simulink model "AlphaIntegrator"  (Simulink 6.6)
settings: Solver=ode45  StartTime=0.0  StopTime=10.0  RelTol=1e-3
values from neighbouring files (symbols this model uses):
  steps = length(canoga_deltaT10)    [CR_init_setup.m]
undefined symbols (not defined in the file or in its folder): alpha, beta, deltat, gamma, iterations
settings Model: Creator=Tommy  LastModifiedBy=Tommy

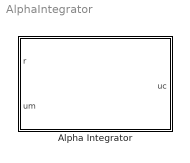
== system AlphaIntegrator ==
  Alpha Integrator : Subsystem
      mask Type: Apha Method with Fixed Number of Iterations
      mask Description: Apha Method with Fixed Number of Iterations

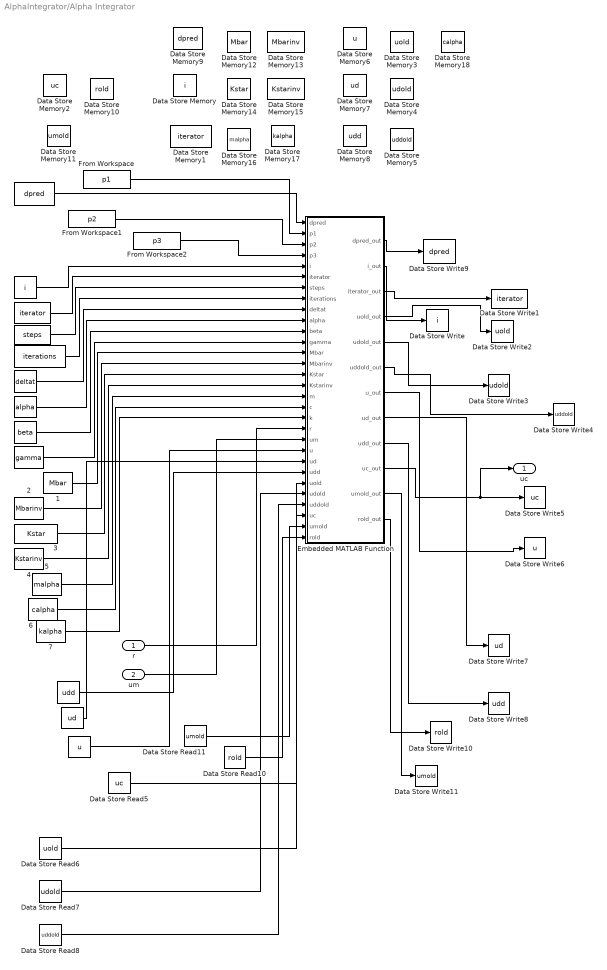
== system AlphaIntegrator/Alpha Integrator ==
  r : Inport
  um : Inport  Port=2
  " " : DataStoreRead  DataStoreName=dpred  SampleTime=1/1024
  "  " : DataStoreRead  DataStoreName=i  SampleTime=1/1024
  "   " : DataStoreRead  DataStoreName=u  SampleTime=1/1024
  "     " : Constant  Value=steps
  "      " : DataStoreRead  DataStoreName=ud  SampleTime=1/1024
  "        " : Constant  Value=alpha
  "            " : Constant  Value=deltat
  "             " : Constant  Value=iterations
  "              " : DataStoreRead  DataStoreName=iterator  SampleTime=1/1024
  "                " : Constant  Value=gamma
  "                 " : DataStoreRead  DataStoreName=udd  SampleTime=1/1024
  "                     " : Constant  Value=beta
  " 1" : DataStoreRead  DataStoreName=Mbar  SampleTime=1/1024
  " 2" : DataStoreRead  DataStoreName=Mbarinv  SampleTime=1/1024
  " 3" : DataStoreRead  DataStoreName=Kstar  SampleTime=1/1024
  " 4" : DataStoreRead  DataStoreName=Kstarinv  SampleTime=1/1024
  " 5" : DataStoreRead  DataStoreName=malpha  SampleTime=1/1024
  " 6" : DataStoreRead  DataStoreName=calpha  SampleTime=1/1024
  " 7" : DataStoreRead  DataStoreName=kalpha  SampleTime=1/1024
  Data Store Memory : DataStoreMemory  DataStoreName=i  InitialValue=0
  Data Store Memory1 : DataStoreMemory  DataStoreName=iterator  InitialValue=0
  Data Store Memory10 : DataStoreMemory  DataStoreName=rold  InitialValue=rold
  Data Store Memory11 : DataStoreMemory  DataStoreName=umold  InitialValue=umold
  Data Store Memory12 : DataStoreMemory  DataStoreName=Mbar  InitialValue=Mbar
  Data Store Memory13 : DataStoreMemory  DataStoreName=Mbarinv  InitialValue=Mbarinv
  Data Store Memory14 : DataStoreMemory  DataStoreName=Kstar  InitialValue=Kstar
  Data Store Memory15 : DataStoreMemory  DataStoreName=Kstarinv  InitialValue=Kstarinv
  Data Store Memory16 : DataStoreMemory  DataStoreName=malpha  InitialValue=malpha
  Data Store Memory17 : DataStoreMemory  DataStoreName=kalpha  InitialValue=kalpha
  Data Store Memory18 : DataStoreMemory  DataStoreName=calpha  InitialValue=calpha
  Data Store Memory2 : DataStoreMemory  DataStoreName=uc  InitialValue=uc
  Data Store Memory3 : DataStoreMemory  DataStoreName=uold  InitialValue=uold
  Data Store Memory4 : DataStoreMemory  DataStoreName=udold  InitialValue=udold
  Data Store Memory5 : DataStoreMemory  DataStoreName=uddold  InitialValue=uddold
  Data Store Memory6 : DataStoreMemory  DataStoreName=u  InitialValue=u
  Data Store Memory7 : DataStoreMemory  DataStoreName=ud  InitialValue=ud
  Data Store Memory8 : DataStoreMemory  DataStoreName=udd  InitialValue=udd
  Data Store Memory9 : DataStoreMemory  DataStoreName=dpred  InitialValue=dpred
  Data Store Read10 : DataStoreRead  DataStoreName=rold  SampleTime=1/1024
  Data Store Read11 : DataStoreRead  DataStoreName=umold  SampleTime=1/1024
  Data Store Read5 : DataStoreRead  DataStoreName=uc  SampleTime=1/1024
  Data Store Read6 : DataStoreRead  DataStoreName=uold  SampleTime=1/1024
  Data Store Read7 : DataStoreRead  DataStoreName=udold  SampleTime=1/1024
  Data Store Read8 : DataStoreRead  DataStoreName=uddold  SampleTime=1/1024
  Data Store Write : DataStoreWrite  DataStoreName=i  SampleTime=1/1024
  Data Store Write1 : DataStoreWrite  DataStoreName=iterator  SampleTime=1/1024
  Data Store Write10 : DataStoreWrite  DataStoreName=rold  SampleTime=1/1024
  Data Store Write11 : DataStoreWrite  DataStoreName=umold  SampleTime=1/1024
  Data Store Write2 : DataStoreWrite  DataStoreName=uold  SampleTime=1/1024
  Data Store Write3 : DataStoreWrite  DataStoreName=udold  SampleTime=1/1024
  Data Store Write4 : DataStoreWrite  DataStoreName=uddold  SampleTime=1/1024
  Data Store Write5 : DataStoreWrite  DataStoreName=uc  SampleTime=1/1024
  Data Store Write6 : DataStoreWrite  DataStoreName=u  SampleTime=1/1024
  Data Store Write7 : DataStoreWrite  DataStoreName=ud  SampleTime=1/1024
  Data Store Write8 : DataStoreWrite  DataStoreName=udd  SampleTime=1/1024
  Data Store Write9 : DataStoreWrite  DataStoreName=dpred  SampleTime=1/1024
  Embedded MATLAB Function : Stateflow chart
  From Workspace : FromWorkspace  VariableName=p1  SampleTime=0
  From Workspace1 : FromWorkspace  VariableName=p2  SampleTime=0
  From Workspace2 : FromWorkspace  VariableName=p3  SampleTime=0
  uc : Outport
  wires:
  Embedded MATLAB Function/1(dpred_out) -> Data Store Write9/1
  Embedded MATLAB Function/3(iterator_out) -> Data Store Write1/1
  Embedded MATLAB Function/2(i_out) -> Data Store Write/1
  " "/1 -> Embedded MATLAB Function/1(dpred)
  "  "/1 -> Embedded MATLAB Function/5(i)
  "              "/1 -> Embedded MATLAB Function/6(iterator)
  "     "/1 -> Embedded MATLAB Function/7(steps)
  "             "/1 -> Embedded MATLAB Function/8(iterations)
  "   "/1 -> Embedded MATLAB Function/22(u)
  "      "/1 -> Embedded MATLAB Function/23(ud)
  "                 "/1 -> Embedded MATLAB Function/24(udd)
  "            "/1 -> Embedded MATLAB Function/9(deltat)
  "                     "/1 -> Embedded MATLAB Function/11(beta)
  " 2"/1 -> Embedded MATLAB Function/14(Mbarinv)
  " 1"/1 -> Embedded MATLAB Function/13(Mbar)
  " 3"/1 -> Embedded MATLAB Function/15(Kstar)
  " 4"/1 -> Embedded MATLAB Function/16(Kstarinv)
  "                "/1 -> Embedded MATLAB Function/12(gamma)
  " 6"/1 -> Embedded MATLAB Function/18(c)
  "        "/1 -> Embedded MATLAB Function/10(alpha)
  " 7"/1 -> Embedded MATLAB Function/19(k)
  r/1 -> Embedded MATLAB Function/20(r)
  Embedded MATLAB Function/5(udold_out) -> Data Store Write3/1
  Embedded MATLAB Function/6(uddold_out) -> Data Store Write4/1
  Data Store Read6/1 -> Embedded MATLAB Function/25(uold)
  Data Store Read7/1 -> Embedded MATLAB Function/26(udold)
  Data Store Read8/1 -> Embedded MATLAB Function/27(uddold)
  um/1 -> Embedded MATLAB Function/21(um)
  Embedded MATLAB Function/10(uc_out) -> Data Store Write5/1, uc/1
  Data Store Read5/1 -> Embedded MATLAB Function/28(uc)
  Embedded MATLAB Function/7(u_out) -> Data Store Write6/1
  Embedded MATLAB Function/8(ud_out) -> Data Store Write7/1
  Embedded MATLAB Function/9(udd_out) -> Data Store Write8/1
  " 5"/1 -> Embedded MATLAB Function/17(m)
  Embedded MATLAB Function/12(rold_out) -> Data Store Write10/1
  Data Store Read10/1 -> Embedded MATLAB Function/30(rold)
  Embedded MATLAB Function/11(umold_out) -> Data Store Write11/1
  Data Store Read11/1 -> Embedded MATLAB Function/29(umold)
  From Workspace/1 -> Embedded MATLAB Function/2(p1)
  From Workspace1/1 -> Embedded MATLAB Function/3(p2)
  From Workspace2/1 -> Embedded MATLAB Function/4(p3)
  Embedded MATLAB Function/4(uold_out) -> Data Store Write2/1

== matlab function Alpha Integrator/Embedded MATLAB Function ==
  data: dpred input inherited; dpred_out output inherited; p1 input inherited; p2 input inherited; p3 input inherited; i input inherited; iterator input inherited; steps input inherited; iterations input inherited; i_out output inherited; iterator_out output inherited; deltat input inherited; alpha input inherited; beta input inherited; gamma input inherited; Mbar input inherited; Mbarinv input inherited; Kstar input inherited; Kstarinv input inherited; m input inherited; c input inherited; k input inherited; r input inherited; um input inherited; u input inherited; ud input inherited; udd input inherited; uold_out output inherited; udold_out output inherited; uddold_out output inherited; u_out output inherited; ud_out output inherited; udd_out output inherited; uold input inherited; udold input inherited; uddold input inherited; uc input inherited; umold input inherited; uc_out output inherited; umold_out output inherited; rold input inherited; rold_out output inherited
function [dpred_out,i_out,iterator_out,uold_out,udold_out,uddold_out,u_out,ud_out,udd_out,uc_out,umold_out,rold_out]  = fcn(dpred,p1,p2,p3,i,iterator,steps,iterations,deltat,alpha,beta,gamma,Mbar,Mbarinv,Kstar,Kstarinv,m,c,k,r,um,u,ud,udd,uold,udold,uddold,uc,umold,rold)
  
%%%%

if (i == 0)
   p11=[p1(1);p2(1);p3(1)];
   udd=inv(m)*(p11-c*ud-k*u);
end

if (i < steps-1)     
    if (iterator == 0)
        i = i + 1;
        pnext=[p1(i+1);p2(i+1);p3(i+1)];pnow=[p1(i);p2(i);p3(i)];
        dpred=[u+deltat*ud+deltat^2*(0.5-beta)*udd]+(deltat^2*beta)*Mbarinv*[(1+alpha)*pnext-alpha*pnow-c*ud-(1+alpha)*(1-gamma)*deltat*c*udd+alpha*rold];        
        uold=u;
        udold=ud;
        uddold=udd;
    end    
    %disp(sprintf('=====\nstep: %i\niterator: %i\np(i): %f\np(i+1): %f\ndpred: %f\nr: %f\nrold: %f\nu: %f\nuc: %f\nud: %f\nudd: %f\num: %f\nuold: %f\nudold: %f\nuddold: %f',i,iterator,p(i),p(i+1),dpred,r,rold,u,uc,ud,udd,um,uold,udold,uddold));
    i_out = i;
    dpred_out = dpred;
    uold_out=uold;
    udold_out=udold;
    uddold_out=uddold;
    uc_out=uc+((dpred-deltat^2*beta*(1+alpha)*Mbarinv*r)-um)/(iterations-iterator);
    rold_out=r;
    umold_out=um;
    if (iterator == 19)
        DELTAd=(-Kstarinv*Mbar*(umold-dpred+deltat^2*beta*(1+alpha)*Mbarinv*rold));
        u=umold+DELTAd;
        rold_out=rold+k*DELTAd;
        udd=(1/(deltat^2*beta))*[u-uold-deltat*udold-deltat^2*(0.5-beta)*uddold];
        ud=udold+deltat*[(1-gamma)*uddold+gamma*udd];
        u_out=u;
        ud_out=ud;
        udd_out=udd;        
        iterator_out = 0;        
    else
        iterator_out = iterator + 1;
        u_out=u;
        ud_out=ud;
        udd_out=udd; 
    end    
else
    dpred_out = dpred;
    i_out = i;
    iterator_out = iterator;
    uold_out=uold;
    udold_out=udold;
    uddold_out=uddold;
    rold_out=rold;
    umold_out=umold;
    uc_out=uc;
    u_out=u;
    ud_out=ud;
    udd_out=udd;    
end
